simulink model "task3_obs"  (R2021b)
settings: Solver=FixedStepAuto  StartTime=0.0  StopTime=20  FixedStep=0.0001  RelTol=1e-3
undefined symbols (not defined in the file): A, C, L1, L2, L3, x0, x0obs
settings Model: Creator=den  LastModifiedBy=den

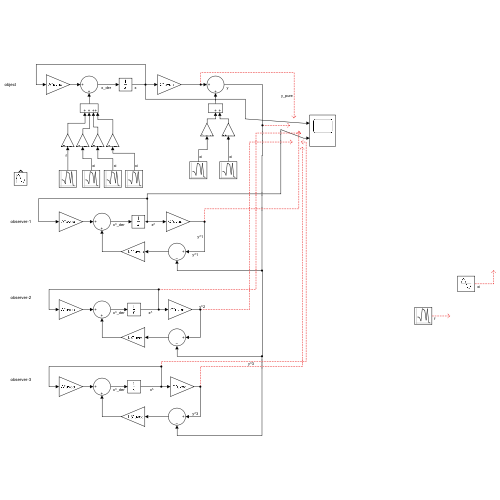
[thumbnail: Simulink's stored preview of the top-level diagram]
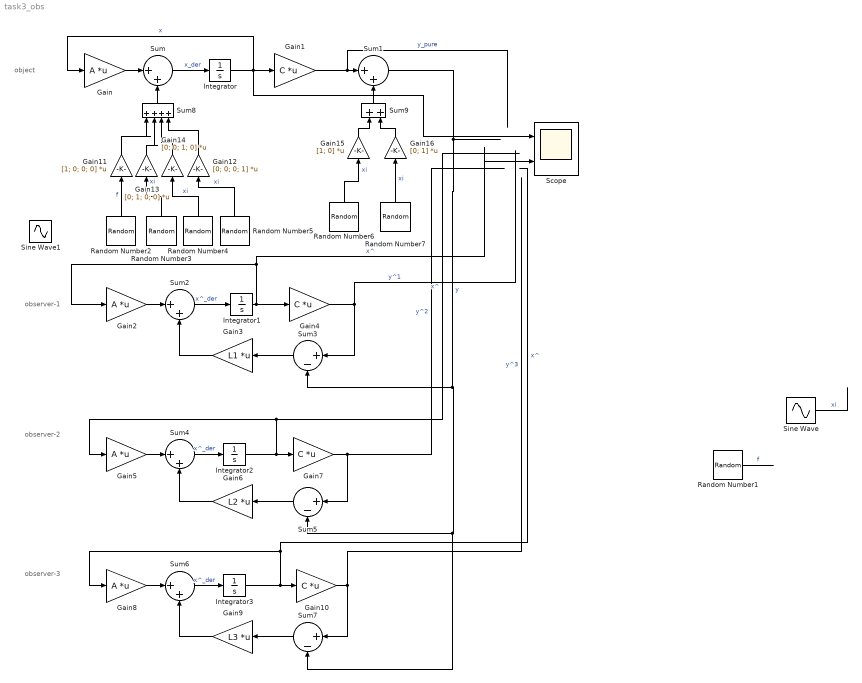
== system task3_obs ==
  note: observer-1
  note: object
  note: observer-2
  note: observer-3
  Gain{,2,5,8} (4 alike) : Gain  Gain=A  Multiplication=Matrix(K*u) (u vector)
  Gain{1,4,7,10} (4 alike) : Gain  Gain=C  Multiplication=Matrix(K*u) (u vector)
  Gain11 : Gain  Gain=[1; 0; 0; 0]  Multiplication=Matrix(K*u) (u vector)
  Gain12 : Gain  Gain=[0; 0; 0; 1]  Multiplication=Matrix(K*u) (u vector)
  Gain13 : Gain  Gain=[0; 1; 0; 0]  Multiplication=Matrix(K*u) (u vector)
  Gain14 : Gain  Gain=[0; 0; 1; 0]  Multiplication=Matrix(K*u) (u vector)
  Gain15 : Gain  Gain=[1; 0]  Multiplication=Matrix(K*u) (u vector)
  Gain16 : Gain  Gain=[0; 1]  Multiplication=Matrix(K*u) (u vector)
  Gain3 : Gain  Gain=L1  Multiplication=Matrix(K*u) (u vector)
  Gain6 : Gain  Gain=L2  Multiplication=Matrix(K*u) (u vector)
  Gain9 : Gain  Gain=L3  Multiplication=Matrix(K*u) (u vector)
  Integrator : Integrator  InitialCondition=x0
  Integrator1 : Integrator  InitialCondition=x0obs
  Integrator2 : Integrator  InitialCondition=x0obs
  Integrator3 : Integrator  InitialCondition=x0obs
  Random Number1 : RandomNumber  Variance=90  Seed=34  SampleTime=0.008
  Random Number2 : RandomNumber  Variance=0.2  Seed=1  SampleTime=0.0005  VectorParams1D=off
  Random Number3 : RandomNumber  Variance=0.2  Seed=2  SampleTime=0.0005  VectorParams1D=off
  Random Number4 : RandomNumber  Variance=0.2  Seed=3  SampleTime=0.0005  VectorParams1D=off
  Random Number5 : RandomNumber  Variance=0.2  Seed=4  SampleTime=0.0005  VectorParams1D=off
  Random Number6 : RandomNumber  Variance=0.2  Seed=5  SampleTime=0.0005
  Random Number7 : RandomNumber  Variance=0.2  Seed=6  SampleTime=0.0005
  Scope : Scope  NumInputPorts=2
  Sine Wave : Sin  Amplitude=5  Bias=0.5  Frequency=8  Phase=pi/3  SampleTime=0
  Sine Wave1 : Sin  Amplitude=79  Bias=-13  Frequency=32  Phase=-pi/2  SampleTime=0
  Sum{,1..2,4,6,9} (6 alike) : Sum  Inputs=|++
  Sum3 : Sum  Inputs=|+-
  Sum5 : Sum  Inputs=|+-
  Sum7 : Sum  Inputs=|+-
  Sum8 : Sum  Inputs=|++++
  wires:
  Gain/1 -> Sum/1
  Sum/1 -> Integrator/1  "x_der"
  Integrator/1 -> Scope/1, Gain1/1, Gain/1  "x"
  Gain1/1 -> Sum1/1  "y_pure"
  Sine Wave/1 -> ?  "xi"
  Gain2/1 -> Sum2/1
  Gain3/1 -> Sum2/2
  Sum2/1 -> Integrator1/1  "x^_der"
  Integrator1/1 -> Scope/2, Gain2/1, Gain4/1  "x^"
  Sum3/1 -> Gain3/1
  Gain4/1 -> Sum3/1  "y^1"
  Random Number1/1 -> ?  "f"
  Sum4/1 -> Integrator2/1  "x^_der"
  Gain7/1 -> Sum5/1  "y^2"
  Integrator2/1 -> Gain7/1, Gain5/1  "x^"
  Gain5/1 -> Sum4/1
  Sum5/1 -> Gain6/1
  Gain6/1 -> Sum4/2
  Sum7/1 -> Gain9/1
  Gain9/1 -> Sum6/2
  Gain8/1 -> Sum6/1
  Gain10/1 -> Sum7/1  "y^3"
  Sum6/1 -> Integrator3/1  "x^_der"
  Integrator3/1 -> Gain8/1, Gain10/1  "x^"
  Sum1/1 -> Sum7/2, Sum5/2, Sum3/2  "y"
  Gain11/1 -> Sum8/1
  Gain13/1 -> Sum8/2
  Gain12/1 -> Sum8/4
  Gain14/1 -> Sum8/3
  Sum9/1 -> Sum1/2
  Gain15/1 -> Sum9/1
  Gain16/1 -> Sum9/2
  Sum8/1 -> Sum/2
  Random Number2/1 -> Gain11/1  "f"
  Random Number6/1 -> Gain15/1  "xi"
  Random Number3/1 -> Gain13/1  "xi"
  Random Number4/1 -> Gain14/1  "xi"
  Random Number5/1 -> Gain12/1  "xi"
  Random Number7/1 -> Gain16/1  "xi"
